simulink model "Carrier_Phase_Shift_2020"  (R2020a)
settings: Solver=VariableStepAuto  StartTime=0.0  StopTime=0.01  MaxStep=1e-7  RelTol=1e-6
InitFcn:
  | fsw=10e3;
  | ma=0.50;
  | ffund=100;
libraries: spsFourierLib x5, spsMeanLib x5
settings Model: Creator=enes_  LastModifiedBy=enes_
settings DataIOCC: SaveFormat=StructureWithTime  ReturnWorkspaceOutputs=off
settings DebuggingCC: SFMachineParentedDataDiag=error

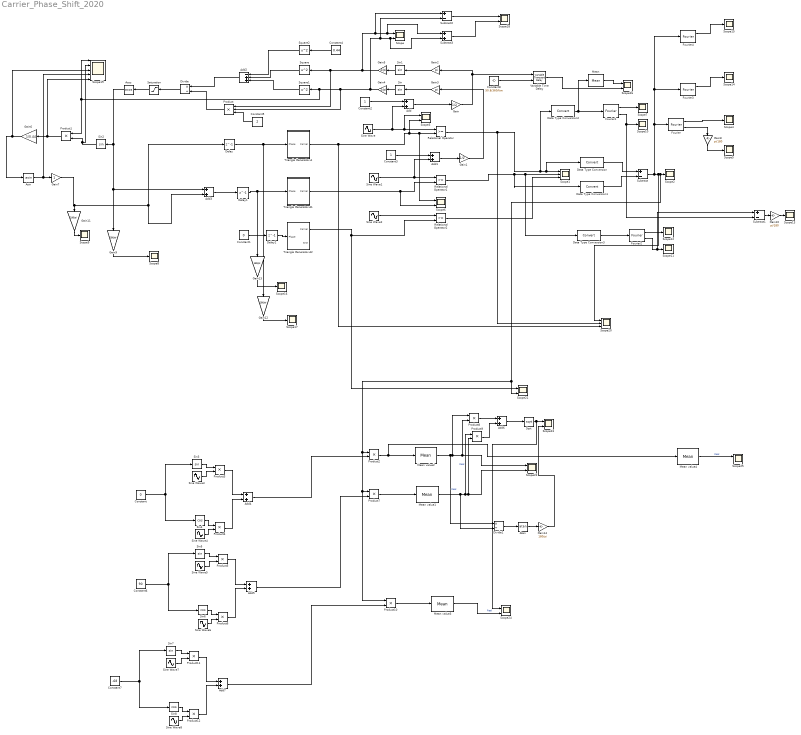
== system Carrier_Phase_Shift_2020 ==
  Acos : Trigonometry  Operator=acos
  Add{,1,3..7} (7 alike) : Sum
  Add2 : Sum  Inputs=-++
  Asin : Trigonometry  Operator=asin
  Atan : Trigonometry  Operator=atan
  Constant : Constant  Value=0
  Constant1 : Constant  Value=0
  Constant2 : Constant
  Constant3 : Constant
  Constant4 : Constant  Value=0.44
  Constant5 : Constant  Value=2
  Constant6 : Constant  Value=90
  Constant7 : Constant  Value=-68
  Constant8 : Constant  Value=50.8/360/fsw
  Data Type Conversion{,1..3} (4 alike) : DataTypeConversion
  Delay : Delay  DelayLength=1
  Delay1 : Delay  DelayLength=1
  Delay2 : Delay  DelayLength=1
  Divide : Product  Inputs=*/
  Divide1 : Product  Inputs=*/
  Fourier : spsFourierLib/Fourier  Freq=fsw  n=1  InInit=[0, 0]  Ts=0
      settings: SourceProductBaseCode=PS
  Fourier1 : spsFourierLib/Fourier  Freq=fsw  n=1  InInit=[0, 0]  Ts=0
      settings: SourceProductBaseCode=PS
  Fourier2 : spsFourierLib/Fourier  Freq=fsw  n=1  InInit=[0, 0]  Ts=0
      settings: SourceProductBaseCode=PS
  Fourier3 : spsFourierLib/Fourier  Freq=ffund  n=102  InInit=[0, 0]  Ts=0
      settings: SourceProductBaseCode=PS
  Fourier4 : spsFourierLib/Fourier  Freq=ffund  n=98  InInit=[0, 0]  Ts=0
      settings: SourceProductBaseCode=PS
  Gain : Gain  Gain=1/2
  Gain1 : Gain  Gain=1/2
  Gain10 : Gain  Gain=pi/180
  Gain{9,11..14} (5 alike) : Gain  Gain=180/pi
  Gain2 : Gain  Gain=pi
  Gain3 : Gain  Gain=pi
  Gain4 : Gain  Gain=2/pi
  Gain5 : Gain  Gain=2/pi
  Gain6 : Gain  Gain=1/0.44
  Gain7 : Gain
  Gain8 : Gain  Gain=pi/180
  Mean : spsMeanLib/Mean  Freq=fsw  Vinit=0  Ts=0
  Mean value1 : spsMeanLib/Mean  Freq=10e3  Vinit=0  Ts=1e-7
  Mean value2 : spsMeanLib/Mean  Freq=10e3  Vinit=0  Ts=1e-7
  Mean value3 : spsMeanLib/Mean  Freq=10e3  Vinit=0  Ts=1e-7
  Mean value4 : spsMeanLib/Mean  Freq=10e3-100  Vinit=0  Ts=1e-7
  Product : Product  Inputs=3
  Product{1..12} (12 alike) : Product
  Relational Operator : RelationalOperator  OutDataTypeStr=boolean  RndMeth=Simplest
  Relational Operator1 : RelationalOperator  OutDataTypeStr=boolean  RndMeth=Simplest
  Relational Operator2 : RelationalOperator  OutDataTypeStr=boolean  RndMeth=Simplest
  Saturation : Saturate  UpperLimit=1  LowerLimit=-1
  Scope{,3,6,18,21..26} (10 alike) : Scope  NumInputPorts=2
  Scope1 : Scope  NumInputPorts=3
  Scope{2,4..5,7..17} (14 alike) : Scope
  Scope19 : Scope  NumInputPorts=5
  Scope20 : Scope  NumInputPorts=3
  Sin{,1..3,5,7} (6 alike) : Trigonometry
  Sin4 : Trigonometry  Operator=cos
  Sin6 : Trigonometry  Operator=cos
  Sin8 : Trigonometry  Operator=cos
  Sine Wave : Sin  Amplitude=ma  Frequency=2*pi*ffund  SampleTime=0
  Sine Wave1 : Sin  Amplitude=ma  Frequency=2*pi*ffund  Phase=2*pi/3  SampleTime=0
  Sine Wave2 : Sin  Amplitude=ma  Frequency=2*pi*ffund  Phase=-2*pi/3  SampleTime=0
  Sine Wave3 : Sin  Frequency=2*pi*fsw  SampleTime=0
  Sine Wave4 : Sin  Frequency=2*pi*fsw  Phase=-pi/2  SampleTime=0
  Sine Wave5 : Sin  Frequency=2*pi*fsw  SampleTime=0
  Sine Wave6 : Sin  Frequency=2*pi*fsw  Phase=-pi/2  SampleTime=0
  Sine Wave7 : Sin  Frequency=2*pi*fsw  SampleTime=0
  Sine Wave8 : Sin  Frequency=2*pi*fsw  Phase=-pi/2  SampleTime=0
  Sqrt : Sqrt  SaturateOnIntegerOverflow=on
  Square : Math  Operator=square  SaturateOnIntegerOverflow=on
  Square1 : Math  Operator=square  SaturateOnIntegerOverflow=on
  Square2 : Math  Operator=square  SaturateOnIntegerOverflow=on
  Subtract : Sum  Inputs=+-
  Subtract1 : Sum  Inputs=+-
  Subtract2 : Sum  Inputs=+-
  Subtract3 : Sum
  Triangle Generator-A : Subsystem
  Triangle Generator-A1 : Subsystem
  Triangle Generator-A2 : Subsystem
  Variable Time Delay : VariableTransportDelay  MaximumDelay=10
  wires:
  Sine Wave/1 -> Add/2, Scope3/1, Relational Operator/1
  Triangle Generator-A/1(Carrier) -> Scope20/3, Scope3/2, Scope6/1, Relational Operator/2
  Triangle Generator-A1/1(Carrier) -> Scope6/2, Relational Operator1/2
  Sine Wave2/1 -> Relational Operator2/1
  Triangle Generator-A2/1(Carrier) -> Scope21/1, Relational Operator2/2
  Constant2/1 -> Add/1
  Add/1 -> Gain/1
  Add1/1 -> Gain1/1
  Constant3/1 -> Add1/1
  Sine Wave1/1 -> Add1/2, Relational Operator1/1
  Relational Operator/1 -> Scope20/2, Data Type Conversion2/1, Data Type Conversion/1, Scope1/1
  Relational Operator1/1 -> Data Type Conversion1/1, Data Type Conversion3/1, Scope1/2
  Relational Operator2/1 -> Scope1/3
  Gain/1 -> Variable Time Delay/1, Gain2/1
  Gain1/1 -> Gain3/1
  Constant4/1 -> Square2/1
  Square2/1 -> Add2/1
  Square/1 -> Add2/2
  Square1/1 -> Add2/3
  Add2/1 -> Divide/1
  Constant5/1 -> Product/3
  Product/1 -> Divide/2
  Divide/1 -> Saturation/1
  Saturation/1 -> Acos/1
  Sin/1 -> Gain4/1
  Sin1/1 -> Gain5/1
  Gain2/1 -> Sin1/1
  Gain3/1 -> Sin/1
  Data Type Conversion/1 -> Subtract/1
  Data Type Conversion1/1 -> Subtract/2
  Fourier/1 -> Scope4/1
  Sin2/1 -> Scope19/2, Product1/2
  Gain4/1 -> Subtract2/2, Subtract3/2, Scope/2, Product/2, Product1/1, Scope19/1, Square1/1
  Product1/1 -> Scope19/5, Gain6/1
  Gain6/1 -> Scope19/3, Asin/1
  Asin/1 -> Scope19/4, Gain7/1
  Constant1/1 -> Delay2/1
  Delay1/1 -> Gain13/1, Triangle Generator-A1/1(Phase)
  Delay2/1 -> Triangle Generator-A2/1(Phase)
  Fourier/2 -> Gain8/1
  Gain8/1 -> Scope5/1
  Add3/1 -> Delay1/1
  Fourier1/1 -> Scope7/1
  Fourier1/2 -> Subtract1/2, Scope10/1
  Data Type Conversion2/1 -> Mean/1, Fourier1/1
  Fourier2/2 -> Subtract1/1, Scope11/1
  Data Type Conversion3/1 -> Fourier2/1
  Fourier2/1 -> Scope12/1
  Subtract1/1 -> Gain10/1
  Gain10/1 -> Scope13/1
  Fourier3/1 -> Scope14/1
  Fourier4/1 -> Scope15/1
  Subtract/1 -> Fourier/1, Fourier4/1, Fourier3/1, Scope20/1, Product10/1, Product7/1, Product2/1, Scope21/2, Scope2/1
  Gain7/1 -> Add3/2, Delay/1, Gain11/1
  Delay/1 -> Triangle Generator-A/1(Phase), Gain12/1
  Gain9/1 -> Scope8/1
  Gain11/1 -> Scope9/1
  Gain12/1 -> Scope17/1
  Subtract2/1 -> Scope18/1
  Subtract3/1 -> Scope18/2
  Gain13/1 -> Scope16/1
  Acos/1 -> Add3/1, Gain9/1, Sin2/1
  Gain5/1 -> Subtract2/1, Subtract3/1, Scope/1, Product/1, Square/1
  Product2/1 -> Mean value4/1, Mean value2/1
  Sine Wave4/1 -> Product4/2
  Product4/1 -> Add4/2
  Product3/1 -> Add4/1
  Constant/1 -> Sin3/1, Sin4/1
  Sin4/1 -> Product4/1
  Sine Wave3/1 -> Product3/2
  Sin3/1 -> Product3/1
  Constant6/1 -> Sin5/1, Sin6/1
  Sine Wave5/1 -> Product5/2
  Sin6/1 -> Product6/1
  Product5/1 -> Add5/1
  Sine Wave6/1 -> Product6/2
  Product6/1 -> Add5/2
  Sin5/1 -> Product5/1
  Add4/1 -> Product2/2
  Add5/1 -> Product7/2
  Product7/1 -> Mean value1/1
  Mean value2/1 -> Divide1/1, Product8/1, Product8/2, Scope22/1  "Real"
  Mean value1/1 -> Divide1/2, Product9/1, Scope22/2, Product9/2  "Real"
  Product8/1 -> Add6/1
  Product9/1 -> Add6/2
  Add6/1 -> Sqrt/1
  Sqrt/1 -> Scope24/1, Scope23/1
  Divide1/1 -> Atan/1
  Atan/1 -> Gain14/1
  Gain14/1 -> Scope23/2
  Product10/1 -> Mean value3/1
  Constant7/1 -> Sin7/1, Sin8/1
  Sine Wave7/1 -> Product11/2
  Sin8/1 -> Product12/1
  Product11/1 -> Add7/1
  Add7/1 -> Product10/2
  Sine Wave8/1 -> Product12/2
  Product12/1 -> Add7/2
  Sin7/1 -> Product11/1
  Mean value3/1 -> Scope24/2  "Real"
  Mean value4/1 -> Scope25/1  "Real"
  Mean/1 -> Scope26/1
  Constant8/1 -> Variable Time Delay/2
  Variable Time Delay/1 -> Scope26/2

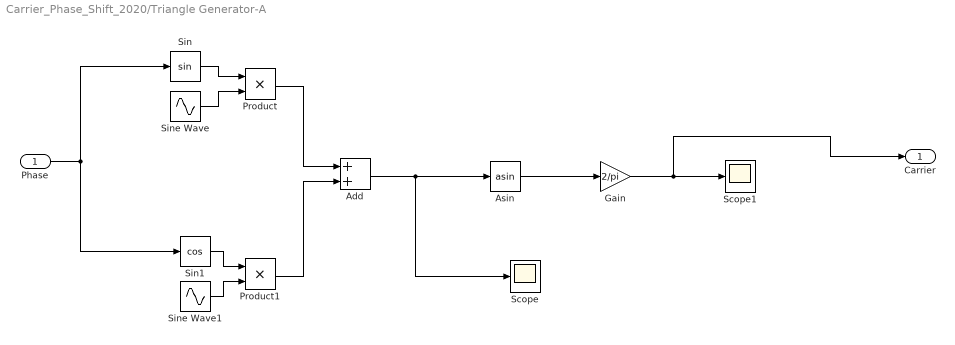
== system Carrier_Phase_Shift_2020/Triangle Generator-A ==
  Phase : Inport
  Add : Sum
  Asin : Trigonometry  Operator=asin
  Gain : Gain  Gain=2/pi
  Product : Product
  Product1 : Product
  Scope : Scope
  Scope1 : Scope
  Sin : Trigonometry
  Sin1 : Trigonometry  Operator=cos
  Sine Wave : Sin  Frequency=2*pi*fsw  SampleTime=0
  Sine Wave1 : Sin  Frequency=2*pi*fsw  Phase=-pi/2  SampleTime=0
  Carrier : Outport
  wires:
  Sin/1 -> Product/1
  Sine Wave/1 -> Product/2
  Phase/1 -> Sin1/1, Sin/1
  Product/1 -> Add/1
  Asin/1 -> Gain/1
  Gain/1 -> Carrier/1, Scope1/1
  Sine Wave1/1 -> Product1/2
  Product1/1 -> Add/2
  Add/1 -> Asin/1, Scope/1
  Sin1/1 -> Product1/1

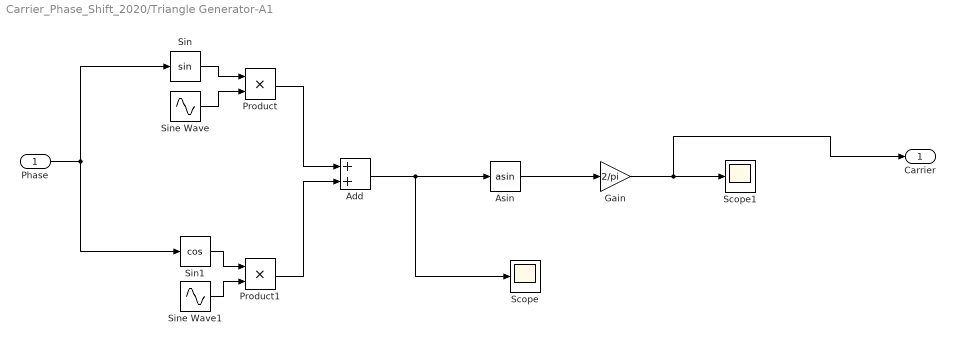
== system Carrier_Phase_Shift_2020/Triangle Generator-A1 ==
  Phase : Inport
  Add : Sum
  Asin : Trigonometry  Operator=asin
  Gain : Gain  Gain=2/pi
  Product : Product
  Product1 : Product
  Scope : Scope
  Scope1 : Scope
  Sin : Trigonometry
  Sin1 : Trigonometry  Operator=cos
  Sine Wave : Sin  Frequency=2*pi*fsw  SampleTime=0
  Sine Wave1 : Sin  Frequency=2*pi*fsw  Phase=-pi/2  SampleTime=0
  Carrier : Outport
  wires:
  Sin/1 -> Product/1
  Sine Wave/1 -> Product/2
  Phase/1 -> Sin1/1, Sin/1
  Product/1 -> Add/1
  Asin/1 -> Gain/1
  Gain/1 -> Carrier/1, Scope1/1
  Sine Wave1/1 -> Product1/2
  Product1/1 -> Add/2
  Add/1 -> Asin/1, Scope/1
  Sin1/1 -> Product1/1

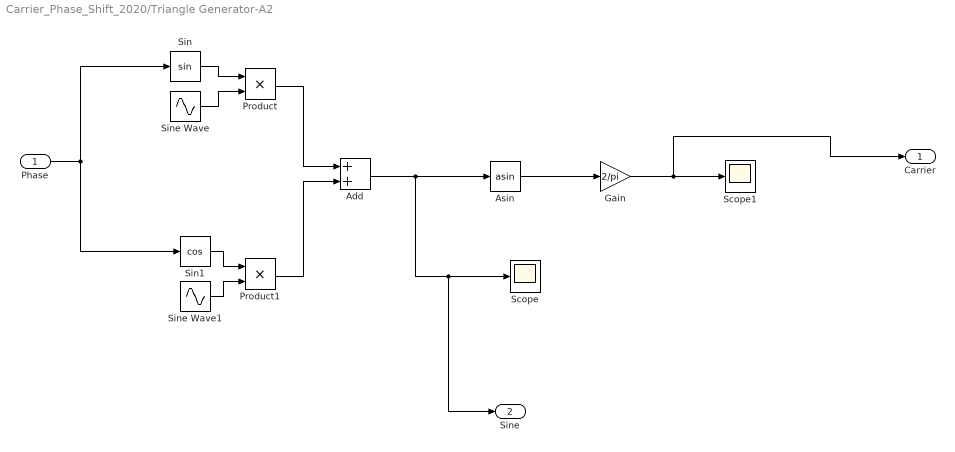
== system Carrier_Phase_Shift_2020/Triangle Generator-A2 ==
  Phase : Inport
  Add : Sum
  Asin : Trigonometry  Operator=asin
  Gain : Gain  Gain=2/pi
  Product : Product
  Product1 : Product
  Scope : Scope
  Scope1 : Scope
  Sin : Trigonometry
  Sin1 : Trigonometry  Operator=cos
  Sine Wave : Sin  Frequency=2*pi*fsw  SampleTime=0
  Sine Wave1 : Sin  Frequency=2*pi*fsw  Phase=-pi/2  SampleTime=0
  Carrier : Outport
  Sine : Outport  Port=2
  wires:
  Sin/1 -> Product/1
  Sine Wave/1 -> Product/2
  Phase/1 -> Sin1/1, Sin/1
  Product/1 -> Add/1
  Asin/1 -> Gain/1
  Gain/1 -> Carrier/1, Scope1/1
  Sine Wave1/1 -> Product1/2
  Product1/1 -> Add/2
  Add/1 -> Asin/1, Sine/1, Scope/1
  Sin1/1 -> Product1/1
